simulink model "simulation_finale"  (R2017a)
settings: Solver=VariableStepAuto  StartTime=0.0  StopTime=1  RelTol=1e-2
InitFcn:
  | variable
values from neighbouring files (symbols this model uses):
  A = (pi*D^2)/4    (= 0.125663706144)    [variable.m]
  a_char_z = 0    [variable.m]
  a_cible_x = 3    [variable.m]
  a_cible_y = 4    [variable.m]
  a_cible_z = 2.22637    [variable.m]
  alpha_phi = pi/4    (= 0.785398163397)    [variable.m]
  alpha_theta = 0    [variable.m]
  Cd = 0.15    [variable.m]
  Cl = 0.05    [variable.m]
  D = 0.4    [variable.m]
  Fc = (294/0.1)*m    (= 14700)    [variable.m]
  g = 9.81    [variable.m]
  m = 5    [variable.m]
  pos_ini_char_z = 0    [variable.m]
  pos_ini_cible_x = 5    [variable.m]
  pos_ini_cible_y = 8    [variable.m]
  pos_ini_cible_z = 5    [variable.m]
  r_missile_canon = 2    [variable.m]
  rho = 1.225    [variable.m]
  v_ini_char_z = 0    [variable.m]
  v_ini_cible_x = 4    [variable.m]
  v_ini_cible_y = 2    [variable.m]
  v_ini_cible_z = 10    [variable.m]
  viscosite = 1.57*10^-5    (= 1.57e-05)    [variable.m]
  w_ini_phi = 1    [variable.m]
  w_ini_theta = 1    [variable.m]
undefined symbols (not defined in the file or in its folder): a_char_x, a_char_y, magnitude, phi_ini_canon, pos_ini_char_x, pos_ini_char_y, theta_ini_canon, v_ini_char_x, v_ini_char_y
settings Model: Creator=stabm1  LastModifiedBy=ahamm2

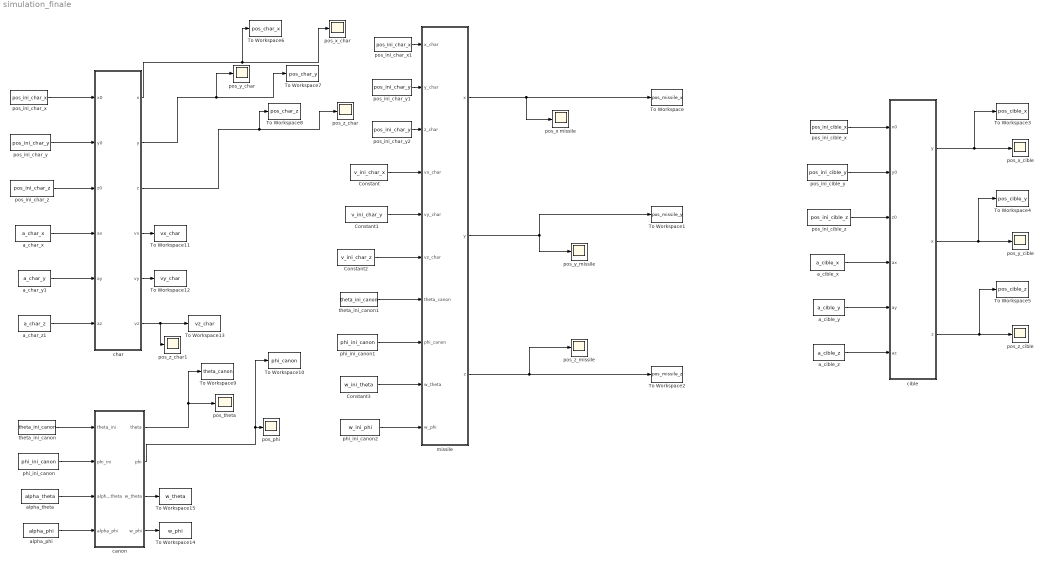
== system simulation_finale ==
  Constant : Constant  Value=v_ini_char_x
  Constant1 : Constant  Value=v_ini_char_y
  Constant2 : Constant  Value=v_ini_char_z
  Constant3 : Constant  Value=w_ini_theta
  To Workspace : ToWorkspace  VariableName=pos_missile_x  SaveFormat=Timeseries  SampleTime=-1
  To Workspace1 : ToWorkspace  VariableName=pos_missile_y  SaveFormat=Timeseries  SampleTime=-1
  To Workspace10 : ToWorkspace  VariableName=phi_canon  SaveFormat=Timeseries  SampleTime=-1
  To Workspace11 : ToWorkspace  VariableName=vx_char  SaveFormat=Timeseries  SampleTime=-1
  To Workspace12 : ToWorkspace  VariableName=vy_char  SaveFormat=Timeseries  SampleTime=-1
  To Workspace13 : ToWorkspace  VariableName=vz_char  SaveFormat=Timeseries  SampleTime=-1
  To Workspace14 : ToWorkspace  VariableName=w_phi  SaveFormat=Timeseries  SampleTime=-1
  To Workspace15 : ToWorkspace  VariableName=w_theta  SaveFormat=Timeseries  SampleTime=-1
  To Workspace2 : ToWorkspace  VariableName=pos_missile_z  SaveFormat=Timeseries  SampleTime=-1
  To Workspace3 : ToWorkspace  VariableName=pos_cible_x  SaveFormat=Timeseries  SampleTime=-1
  To Workspace4 : ToWorkspace  VariableName=pos_cible_y  SaveFormat=Timeseries  SampleTime=-1
  To Workspace5 : ToWorkspace  VariableName=pos_cible_z  SaveFormat=Timeseries  SampleTime=-1
  To Workspace6 : ToWorkspace  VariableName=pos_char_x  SaveFormat=Timeseries  SampleTime=-1
  To Workspace7 : ToWorkspace  VariableName=pos_char_y  SaveFormat=Timeseries  SampleTime=-1
  To Workspace8 : ToWorkspace  VariableName=pos_char_z  SaveFormat=Timeseries  SampleTime=-1
  To Workspace9 : ToWorkspace  VariableName=theta_canon  SaveFormat=Timeseries  SampleTime=-1
  a_char_x : Constant  Value=a_char_x
  a_char_y1 : Constant  Value=a_char_y
  a_char_z1 : Constant  Value=a_char_z
  a_cible_x : Constant  Value=a_cible_x
  a_cible_y : Constant  Value=a_cible_y
  a_cible_z : Constant  Value=a_cible_z
  alpha_phi : Constant  Value=alpha_phi
  alpha_theta : Constant  Value=alpha_theta
  canon : Subsystem  TreatAsAtomicUnit=on
  char : Subsystem  TreatAsAtomicUnit=on
  cible : Subsystem  TreatAsAtomicUnit=on
  missile : Subsystem  TreatAsAtomicUnit=on
  phi_ini_canon : Constant  Value=phi_ini_canon
  phi_ini_canon1 : Constant  Value=phi_ini_canon
  phi_ini_canon2 : Constant  Value=w_ini_phi
  pos_ini_char_x : Constant  Value=pos_ini_char_x
  pos_ini_char_x1 : Constant  Value=pos_ini_char_x
  pos_ini_char_y : Constant  Value=pos_ini_char_y
  pos_ini_char_y1 : Constant  Value=pos_ini_char_y
  pos_ini_char_y2 : Constant  Value=pos_ini_char_y
  pos_ini_char_z : Constant  Value=pos_ini_char_z
  pos_ini_cible_x : Constant  Value=pos_ini_cible_x
  pos_ini_cible_y : Constant  Value=pos_ini_cible_y
  pos_ini_cible_z : Constant  Value=pos_ini_cible_z
  pos_phi : Scope
  pos_theta : Scope
  pos_x missile : Scope
  pos_x_char : Scope
  pos_x_cible : Scope
  pos_y_char : Scope
  pos_y_cible : Scope
  pos_y_missile : Scope
  pos_z_char : Scope
  pos_z_char1 : Scope
  pos_z_cible : Scope
  pos_z_missile : Scope
  theta_ini_canon : Constant  Value=theta_ini_canon
  theta_ini_canon1 : Constant  Value=theta_ini_canon
  wires:
  a_char_y1/1 -> char/5(ay)
  a_char_z1/1 -> char/6(az)
  a_char_x/1 -> char/4(ax)
  a_cible_y/1 -> cible/5(ay)
  cible/1(y) -> To Workspace3/1, pos_x_cible/1
  a_cible_x/1 -> cible/4(ax)
  a_cible_z/1 -> cible/6(az)
  pos_ini_cible_z/1 -> cible/3(z0)
  pos_ini_cible_y/1 -> cible/2(y0)
  cible/3(z) -> To Workspace5/1, pos_z_cible/1
  pos_ini_cible_x/1 -> cible/1(x0)
  cible/2(x) -> To Workspace4/1, pos_y_cible/1
  theta_ini_canon/1 -> canon/1(theta_ini)
  alpha_phi/1 -> canon/4(alpha_phi)
  alpha_theta/1 -> canon/3(alpha_theta)
  phi_ini_canon/1 -> canon/2(phi_ini)
  missile/1(x) -> To Workspace/1, pos_x missile/1
  missile/2(y) -> To Workspace1/1, pos_y_missile/1
  missile/3(z) -> pos_z_missile/1, To Workspace2/1
  char/1(x) -> pos_x_char/1, To Workspace6/1
  char/2(y) -> pos_y_char/1, To Workspace7/1
  char/3(z) -> To Workspace8/1, pos_z_char/1
  canon/1(theta) -> pos_theta/1, To Workspace9/1
  canon/2(phi) -> pos_phi/1, To Workspace10/1
  pos_ini_char_x/1 -> char/1(x0)
  pos_ini_char_y/1 -> char/2(y0)
  pos_ini_char_z/1 -> char/3(z0)
  pos_ini_char_x1/1 -> missile/1(x_char)
  pos_ini_char_y1/1 -> missile/2(y_char)
  pos_ini_char_y2/1 -> missile/3(z_char)
  Constant/1 -> missile/4(vx_char)
  Constant1/1 -> missile/5(vy_char)
  Constant2/1 -> missile/6(vz_char)
  char/4(vx) -> To Workspace11/1
  char/5(vy) -> To Workspace12/1
  char/6(vz) -> pos_z_char1/1, To Workspace13/1
  theta_ini_canon1/1 -> missile/7(theta_canon)
  phi_ini_canon1/1 -> missile/8(phi_canon)
  Constant3/1 -> missile/9(w_theta)
  phi_ini_canon2/1 -> missile/10(w_phi)
  canon/3(w_theta) -> To Workspace15/1
  canon/4(w_phi) -> To Workspace14/1

== system simulation_finale/canon ==
  theta_ini : Inport
  phi_ini : Inport  Port=2
  alpha_theta : Inport  Port=3
  alpha_phi : Inport  Port=4
  angle_theta : Subsystem  TreatAsAtomicUnit=on
  angle_theta1 : Subsystem  TreatAsAtomicUnit=on
  theta : Outport
  phi : Outport  Port=2
  w_theta : Outport  Port=3
  w_phi : Outport  Port=4
  wires:
  theta_ini/1 -> angle_theta/1(theta_ini)
  alpha_theta/1 -> angle_theta/2(alpha_theta)
  angle_theta/1(theta) -> theta/1
  angle_theta1/1(phi) -> phi/1
  alpha_phi/1 -> angle_theta1/2(alpha_phi)
  phi_ini/1 -> angle_theta1/1(phi_ini)
  angle_theta1/2(w_phi) -> w_phi/1
  angle_theta/2(w_theta) -> w_theta/1

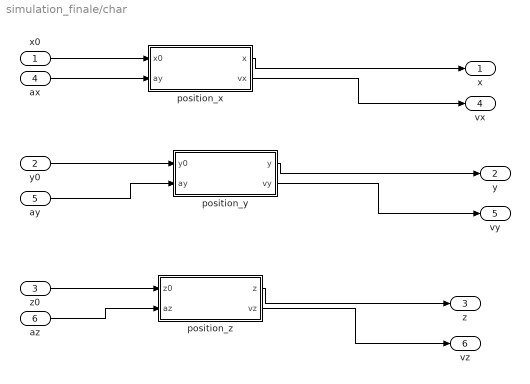
== system simulation_finale/char ==
  x0 : Inport
  y0 : Inport  Port=2
  z0 : Inport  Port=3
  ax : Inport  Port=4
  ay : Inport  Port=5
  az : Inport  Port=6
  position_x : Subsystem  TreatAsAtomicUnit=on
  position_y : Subsystem  TreatAsAtomicUnit=on
  position_z : Subsystem  TreatAsAtomicUnit=on
  x : Outport
  y : Outport  Port=2
  z : Outport  Port=3
  vx : Outport  Port=4
  vy : Outport  Port=5
  vz : Outport  Port=6
  wires:
  x0/1 -> position_x/1(x0)
  ax/1 -> position_x/2(ay)
  position_x/1(x) -> x/1
  y0/1 -> position_y/1(y0)
  ay/1 -> position_y/2(ay)
  position_y/1(y) -> y/1
  z0/1 -> position_z/1(z0)
  az/1 -> position_z/2(az)
  position_z/1(z) -> z/1
  position_x/2(vx) -> vx/1
  position_y/2(vy) -> vy/1
  position_z/2(vz) -> vz/1

== system simulation_finale/cible ==
  note: r = r0+v*t+at^2
  x0 : Inport
  y0 : Inport  Port=2
  z0 : Inport  Port=3
  ax : Inport  Port=4
  ay : Inport  Port=5
  az : Inport  Port=6
  position_x : Subsystem  TreatAsAtomicUnit=on
  position_y : Subsystem  TreatAsAtomicUnit=on
  position_z : Subsystem  TreatAsAtomicUnit=on
  y : Outport
  x : Outport  Port=2
  z : Outport  Port=3
  wires:
  x0/1 -> position_x/1(x0)
  ax/1 -> position_x/2(ay)
  position_x/1(x) -> x/1
  y0/1 -> position_y/1(y0)
  ay/1 -> position_y/2(ay)
  position_y/1(y) -> y/1
  z0/1 -> position_z/1(z0)
  az/1 -> position_z/2(az)
  position_z/1(z) -> z/1

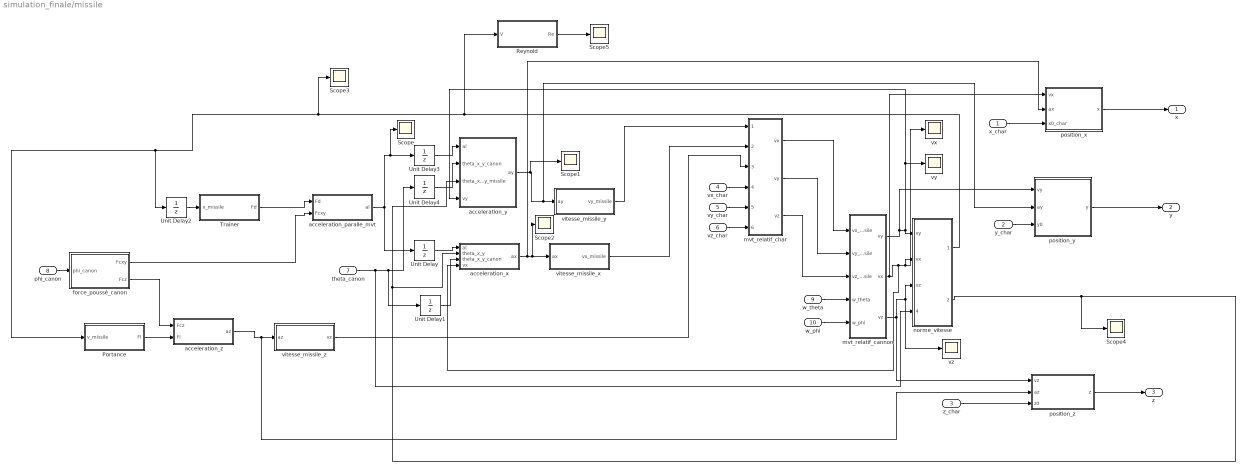
== system simulation_finale/missile ==
  x_char : Inport
  y_char : Inport  Port=2
  z_char : Inport  Port=3
  vx_char : Inport  Port=4
  vy_char : Inport  Port=5
  vz_char : Inport  Port=6
  theta_canon : Inport  Port=7
  phi_canon : Inport  Port=8
  w_theta : Inport  Port=9
  w_phi : Inport  Port=10
  Portance : Subsystem  TreatAsAtomicUnit=on
  Reynold : Subsystem  TreatAsAtomicUnit=on
  Scope{,1..5} (6 alike) : Scope
  Trainer : Subsystem  TreatAsAtomicUnit=on
  Unit Delay{,1..4} (5 alike) : UnitDelay  SampleTime=-1
  acceleration_paralle_mvt : Subsystem  TreatAsAtomicUnit=on
  acceleration_x : Subsystem  TreatAsAtomicUnit=on
  acceleration_y : Subsystem  TreatAsAtomicUnit=on
  acceleration_z : Subsystem  TreatAsAtomicUnit=on
  force_poussé_canon : Subsystem  TreatAsAtomicUnit=on
  mvt_relatif_cannon : Subsystem  TreatAsAtomicUnit=on
  mvt_relatif_char : Subsystem  TreatAsAtomicUnit=on
  "norme_vitesse " : Subsystem  TreatAsAtomicUnit=on
  position_x : Subsystem  TreatAsAtomicUnit=on
  position_y : Subsystem  TreatAsAtomicUnit=on
  position_z : Subsystem  TreatAsAtomicUnit=on
  vitesse_missile_x : Subsystem  TreatAsAtomicUnit=on
  vitesse_missile_y : Subsystem  TreatAsAtomicUnit=on
  vitesse_missile_z : Subsystem  TreatAsAtomicUnit=on
  vx : Scope
  vy : Scope
  vz : Scope
  x : Outport
  y : Outport  Port=2
  z : Outport  Port=3
  wires:
  Trainer/1(Fd) -> acceleration_paralle_mvt/1(Fd)
  Portance/1(Fl) -> acceleration_z/2(Fl)
  acceleration_paralle_mvt/1(al) -> Scope/1, Unit Delay3/1, Unit Delay/1
  "norme_vitesse "/1(v_missile) -> Reynold/1(V), Scope3/1, Unit Delay2/1, Portance/1(v_missile)
  Unit Delay/1 -> acceleration_x/1(al)
  Unit Delay2/1 -> Trainer/1(v_missile)
  Unit Delay3/1 -> acceleration_y/1(al)
  Unit Delay4/1 -> acceleration_y/2(theta_x_y_canon)
  phi_canon/1 -> force_poussé_canon/1(phi_canon)
  force_poussé_canon/2(Fcz) -> acceleration_z/1(Fcz)
  force_poussé_canon/1(Fcxy) -> acceleration_paralle_mvt/2(Fcxy)
  mvt_relatif_cannon/3(vz) -> position_z/1(vz), vz/1, "norme_vitesse "/3(vz)
  mvt_relatif_cannon/1(vy) -> position_y/1(vy), acceleration_y/4(vy), vy/1, "norme_vitesse "/1(vy)
  vitesse_missile_z/1(vz) -> mvt_relatif_char/3(vz_missile)
  position_y/1(y) -> y/1
  position_z/1(z) -> z/1
  position_x/1(x) -> x/1
  z_char/1 -> position_z/3(z0)
  x_char/1 -> position_x/3(x0_char)
  y_char/1 -> position_y/3(y0)
  vitesse_missile_y/1(vy_missile) -> mvt_relatif_char/1(vy_missile)
  acceleration_z/1(az) -> position_z/2(az), vitesse_missile_z/1(az)
  vx_char/1 -> mvt_relatif_char/4(vx_char)
  vy_char/1 -> mvt_relatif_char/5(vy_char)
  vz_char/1 -> mvt_relatif_char/6(vz_char)
  vitesse_missile_x/1(vx_missile) -> mvt_relatif_char/2(vx_missile)
  w_theta/1 -> mvt_relatif_cannon/4(w_theta)
  w_phi/1 -> mvt_relatif_cannon/5(w_phi)
  mvt_relatif_char/3(vz) -> mvt_relatif_cannon/3(vz_missile)
  mvt_relatif_char/2(vy) -> mvt_relatif_cannon/2(vy_missile)
  mvt_relatif_char/1(vx) -> mvt_relatif_cannon/1(vx_missile)
  "norme_vitesse "/2(theta_x_y) -> Scope4/1, acceleration_x/2(theta_x_y), acceleration_y/3(theta_x_y_missile)
  Unit Delay1/1 -> acceleration_x/3(theta_x_y_canon)
  theta_canon/1 -> "norme_vitesse "/4(theta_canon), Unit Delay1/1, Unit Delay4/1
  Reynold/1(Re) -> Scope5/1
  acceleration_x/1(ax) -> vitesse_missile_x/1(ax), Scope2/1, position_x/2(ax)
  acceleration_y/1(ay) -> Scope1/1, position_y/2(ay), vitesse_missile_y/1(ay)
  mvt_relatif_cannon/2(vx) -> acceleration_x/4(vx), vx/1, "norme_vitesse "/2(vx), position_x/1(vx)

== system simulation_finale/canon/angle_theta ==
  theta_ini : Inport
  alpha_theta : Inport  Port=2
  Add : Sum
  Add1 : Sum
  Clock : Clock
  Gain : Gain  Gain=1/2
  Math Function : Math  Operator=magnitude^2  SaturateOnIntegerOverflow=on
  Product : Product
  Product1 : Product
  v : Integrator  InitialCondition=w_ini_theta
  theta : Outport
  w_theta : Outport  Port=2
  wires:
  Add1/1 -> theta/1
  Math Function/1 -> Product1/1
  Product/1 -> Add/2
  Add/1 -> Add1/1
  alpha_theta/1 -> Product1/2, v/1
  Clock/1 -> Math Function/1, Product/2
  theta_ini/1 -> Add/1
  Gain/1 -> Add1/2
  Product1/1 -> Gain/1
  v/1 -> w_theta/1, Product/1

== system simulation_finale/canon/angle_theta1 ==
  phi_ini : Inport
  alpha_phi : Inport  Port=2
  Add : Sum
  Add1 : Sum
  Clock : Clock
  Gain : Gain  Gain=1/2
  Math Function : Math  Operator=magnitude^2  SaturateOnIntegerOverflow=on
  Product : Product
  Product1 : Product
  v : Integrator  InitialCondition=w_ini_phi
  phi : Outport
  w_phi : Outport  Port=2
  wires:
  Add1/1 -> phi/1
  Math Function/1 -> Product1/1
  Product/1 -> Add/2
  Add/1 -> Add1/1
  alpha_phi/1 -> Product1/2, v/1
  Clock/1 -> Math Function/1, Product/2
  phi_ini/1 -> Add/1
  Gain/1 -> Add1/2
  Product1/1 -> Gain/1
  v/1 -> w_phi/1, Product/1

== system simulation_finale/char/position_x ==
  x0 : Inport
  ay : Inport  Port=2
  Add : Sum
  Add1 : Sum
  Clock : Clock
  Gain : Gain  Gain=1/2
  Math Function : Math  Operator=magnitude^2  SaturateOnIntegerOverflow=on
  Product : Product
  Product1 : Product
  v : Integrator  InitialCondition=v_ini_char_x
  x : Outport
  vx : Outport  Port=2
  wires:
  v/1 -> vx/1, Product/1
  Product/1 -> Add/2
  Math Function/1 -> Product1/1
  Add/1 -> Add1/1
  Product1/1 -> Gain/1
  Gain/1 -> Add1/2
  Clock/1 -> Math Function/1, Product/2
  x0/1 -> Add/1
  ay/1 -> Product1/2, v/1
  Add1/1 -> x/1

== system simulation_finale/char/position_y ==
  y0 : Inport
  ay : Inport  Port=2
  Add : Sum
  Add1 : Sum
  Clock : Clock
  Gain : Gain  Gain=1/2
  Math Function : Math  Operator=magnitude^2  SaturateOnIntegerOverflow=on
  Product : Product
  Product1 : Product
  v : Integrator  InitialCondition=v_ini_char_y
  y : Outport
  vy : Outport  Port=2
  wires:
  v/1 -> vy/1, Product/1
  Product/1 -> Add/2
  Math Function/1 -> Product1/1
  Add/1 -> Add1/1
  Product1/1 -> Gain/1
  Gain/1 -> Add1/2
  Clock/1 -> Math Function/1, Product/2
  y0/1 -> Add/1
  ay/1 -> Product1/2, v/1
  Add1/1 -> y/1

== system simulation_finale/char/position_z ==
  z0 : Inport
  az : Inport  Port=2
  Add : Sum
  Add1 : Sum
  Clock : Clock
  Gain : Gain  Gain=1/2
  Math Function : Math  Operator=magnitude^2  SaturateOnIntegerOverflow=on
  Product : Product
  Product1 : Product
  v : Integrator  InitialCondition=v_ini_char_z
  z : Outport
  vz : Outport  Port=2
  wires:
  v/1 -> Product/1, vz/1
  Product/1 -> Add/2
  Math Function/1 -> Product1/1
  Add/1 -> Add1/1
  Product1/1 -> Gain/1
  Gain/1 -> Add1/2
  Clock/1 -> Math Function/1, Product/2
  z0/1 -> Add/1
  az/1 -> Product1/2, v/1
  Add1/1 -> z/1

== system simulation_finale/cible/position_x ==
  x0 : Inport
  ay : Inport  Port=2
  Add : Sum
  Add1 : Sum
  Clock : Clock
  Gain : Gain  Gain=1/2
  Math Function : Math  Operator=magnitude^2  SaturateOnIntegerOverflow=on
  Product : Product
  Product1 : Product
  v : Integrator  InitialCondition=v_ini_cible_x
  x : Outport
  wires:
  v/1 -> Product/1
  Product/1 -> Add/2
  Math Function/1 -> Product1/1
  Add/1 -> Add1/1
  Product1/1 -> Gain/1
  Gain/1 -> Add1/2
  Clock/1 -> Math Function/1, Product/2
  x0/1 -> Add/1
  ay/1 -> Product1/2, v/1
  Add1/1 -> x/1

== system simulation_finale/cible/position_y ==
  y0 : Inport
  ay : Inport  Port=2
  Add : Sum
  Add1 : Sum
  Clock : Clock
  Gain : Gain  Gain=1/2
  Math Function : Math  Operator=magnitude^2  SaturateOnIntegerOverflow=on
  Product : Product
  Product1 : Product
  v : Integrator  InitialCondition=v_ini_cible_y
  y : Outport
  wires:
  v/1 -> Product/1
  Product/1 -> Add/2
  Math Function/1 -> Product1/1
  Add/1 -> Add1/1
  Product1/1 -> Gain/1
  Gain/1 -> Add1/2
  Clock/1 -> Math Function/1, Product/2
  y0/1 -> Add/1
  ay/1 -> Product1/2, v/1
  Add1/1 -> y/1

== system simulation_finale/cible/position_z ==
  z0 : Inport
  az : Inport  Port=2
  Add : Sum
  Add1 : Sum
  Clock : Clock
  Gain : Gain  Gain=1/2
  Math Function : Math  Operator=magnitude^2  SaturateOnIntegerOverflow=on
  Product : Product
  Product1 : Product
  v : Integrator  InitialCondition=v_ini_cible_z
  z : Outport
  wires:
  v/1 -> Product/1
  Product/1 -> Add/2
  Math Function/1 -> Product1/1
  Add/1 -> Add1/1
  Product1/1 -> Gain/1
  Gain/1 -> Add1/2
  Clock/1 -> Math Function/1, Product/2
  z0/1 -> Add/1
  az/1 -> Product1/2, v/1
  Add1/1 -> z/1

== system simulation_finale/missile/Portance ==
  v_missile : Inport
  Constant : Constant  Value=Cl
  Gain : Gain  Gain=0.5*rho*A
  Math Function : Math  Operator=magnitude^2  SaturateOnIntegerOverflow=on
  Product : Product
  Fl : Outport
  wires:
  Product/1 -> Fl/1
  Gain/1 -> Product/1
  Constant/1 -> Product/2
  v_missile/1 -> Math Function/1
  Math Function/1 -> Gain/1

== system simulation_finale/missile/Reynold ==
  V : Inport
  Gain : Gain  Gain=D/viscosite
  To Workspace : ToWorkspace  VariableName=Re  SaveFormat=Timeseries  SampleTime=-1
  Re : Outport
  wires:
  V/1 -> Gain/1
  Gain/1 -> Re/1, To Workspace/1

== system simulation_finale/missile/Trainer ==
  v_missile : Inport
  Constant : Constant  Value=Cd
  Gain : Gain  Gain=0.5*rho*A
  Math Function : Math  Operator=magnitude^2  SaturateOnIntegerOverflow=on
  Product : Product
  Fd : Outport
  wires:
  v_missile/1 -> Math Function/1
  Math Function/1 -> Gain/1
  Gain/1 -> Product/1
  Constant/1 -> Product/2
  Product/1 -> Fd/1

== system simulation_finale/missile/acceleration_paralle_mvt ==
  Fd : Inport
  Fcxy : Inport  Port=2
  Add : Sum  Inputs=-+
  Gain : Gain  Gain=1/m
  al : Outport
  wires:
  Gain/1 -> al/1
  Add/1 -> Gain/1
  Fcxy/1 -> Add/2
  Fd/1 -> Add/1

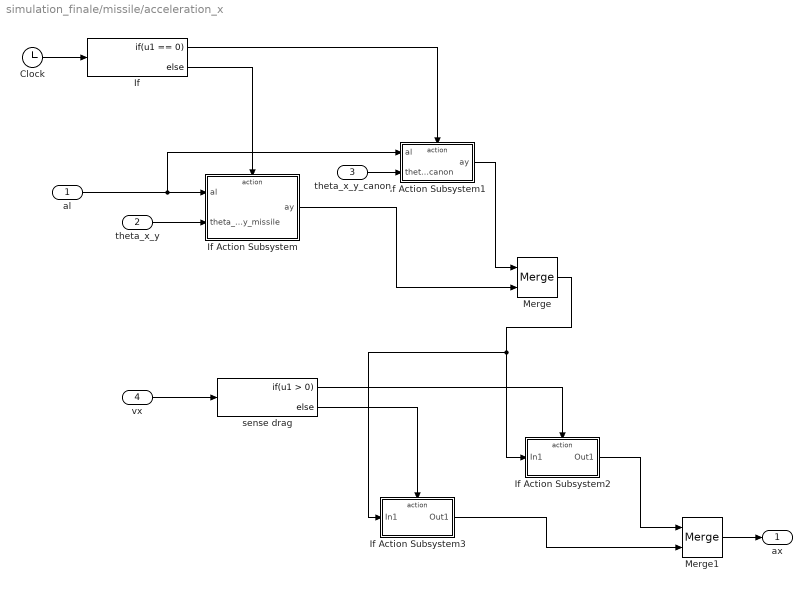
== system simulation_finale/missile/acceleration_x ==
  al : Inport
  theta_x_y : Inport  Port=2
  theta_x_y_canon : Inport  Port=3
  vx : Inport  Port=4
  Clock : Clock
  If : If  IfExpression=u1 == 0
  If Action Subsystem : Subsystem  TreatAsAtomicUnit=on
  If Action Subsystem1 : Subsystem  TreatAsAtomicUnit=on
  If Action Subsystem2 : Subsystem  TreatAsAtomicUnit=on
  If Action Subsystem3 : Subsystem  TreatAsAtomicUnit=on
  Merge : Merge
  Merge1 : Merge
  sense drag : If  ZeroCross=off
  ax : Outport
  wires:
  If/1 -> If Action Subsystem1/Action
  theta_x_y/1 -> If Action Subsystem/2(theta_x_y_missile)
  If Action Subsystem/1(ay) -> Merge/2
  If/2 -> If Action Subsystem/Action
  theta_x_y_canon/1 -> If Action Subsystem1/2(theta_canon)
  Clock/1 -> If/1
  al/1 -> If Action Subsystem1/1(al), If Action Subsystem/1(al)
  If Action Subsystem1/1(ay) -> Merge/1
  sense drag/1 -> If Action Subsystem2/Action
  sense drag/2 -> If Action Subsystem3/Action
  Merge1/1 -> ax/1
  If Action Subsystem2/1(Out1) -> Merge1/1
  If Action Subsystem3/1(Out1) -> Merge1/2
  Merge/1 -> If Action Subsystem3/1(In1), If Action Subsystem2/1(In1)
  vx/1 -> sense drag/1

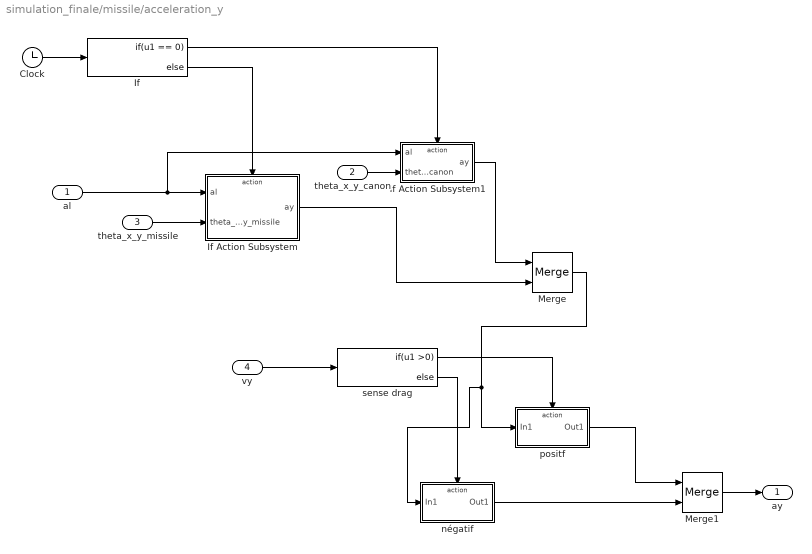
== system simulation_finale/missile/acceleration_y ==
  al : Inport
  theta_x_y_canon : Inport  Port=2
  theta_x_y_missile : Inport  Port=3
  vy : Inport  Port=4
  Clock : Clock
  If : If  IfExpression=u1 == 0
  If Action Subsystem : Subsystem  TreatAsAtomicUnit=on
  If Action Subsystem1 : Subsystem  TreatAsAtomicUnit=on
  Merge : Merge
  Merge1 : Merge
  négatif : Subsystem  TreatAsAtomicUnit=on
  positf : Subsystem  TreatAsAtomicUnit=on
  sense drag : If  IfExpression=u1 >0  ZeroCross=off
  ay : Outport
  wires:
  If/1 -> If Action Subsystem1/Action
  If/2 -> If Action Subsystem/Action
  Clock/1 -> If/1
  If Action Subsystem1/1(ay) -> Merge/1
  al/1 -> If Action Subsystem1/1(al), If Action Subsystem/1(al)
  theta_x_y_canon/1 -> If Action Subsystem1/2(theta_canon)
  If Action Subsystem/1(ay) -> Merge/2
  theta_x_y_missile/1 -> If Action Subsystem/2(theta_x_y_missile)
  vy/1 -> sense drag/1
  Merge1/1 -> ay/1
  sense drag/1 -> positf/Action
  sense drag/2 -> négatif/Action
  Merge/1 -> négatif/1(In1), positf/1(In1)
  positf/1(Out1) -> Merge1/1
  négatif/1(Out1) -> Merge1/2

== system simulation_finale/missile/acceleration_z ==
  Fcz : Inport
  Fl : Inport  Port=2
  Add : Sum  Inputs=++-
  Constant : Constant  Value=m*g
  Gain : Gain  Gain=1/m
  Scope : Scope
  Scope1 : Scope
  Scope2 : Scope
  az : Outport
  wires:
  Fl/1 -> Scope/1, Add/1
  Add/1 -> Gain/1
  Gain/1 -> az/1
  Constant/1 -> Scope1/1, Add/3
  Fcz/1 -> Scope2/1, Add/2

== system simulation_finale/missile/force_poussé_canon ==
  phi_canon : Inport
  Clock : Clock
  If : If  IfExpression=u1 ==0  ZeroCross=off
  Merge : Merge
  Merge1 : Merge
  pas de poussé : Subsystem  TreatAsAtomicUnit=on
  poussé du canon : Subsystem  TreatAsAtomicUnit=on
  Fcxy : Outport
  Fcz : Outport  Port=2
  wires:
  Clock/1 -> If/1
  Merge/1 -> Fcz/1
  Merge1/1 -> Fcxy/1
  If/1 -> poussé du canon/Action
  phi_canon/1 -> poussé du canon/1(phi_canon)
  poussé du canon/1(Fcz) -> Merge/1
  poussé du canon/2(Fcxy) -> Merge1/1
  If/2 -> pas de poussé/Action
  pas de poussé/1(pas_de_pousse) -> Merge/2
  pas de poussé/2(pas_de_pousse2) -> Merge1/2

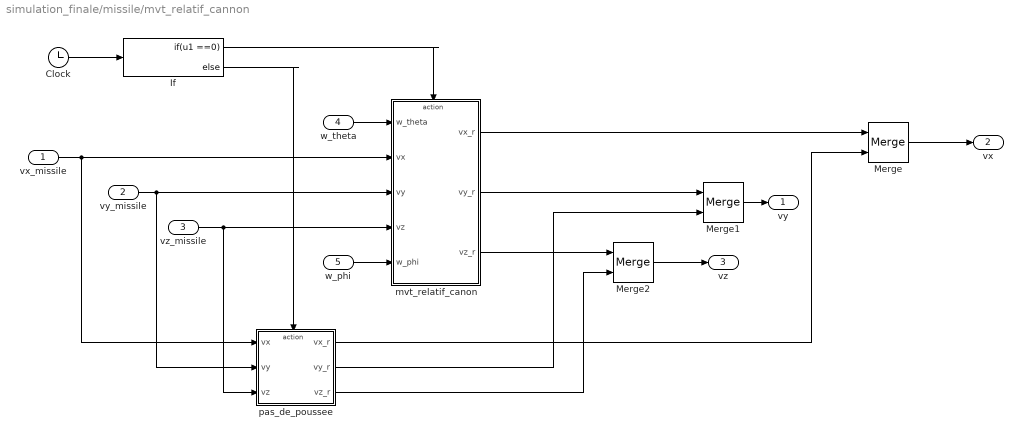
== system simulation_finale/missile/mvt_relatif_cannon ==
  vx_missile : Inport
  vy_missile : Inport  Port=2
  vz_missile : Inport  Port=3
  w_theta : Inport  Port=4
  w_phi : Inport  Port=5
  Clock : Clock
  If : If  IfExpression=u1 ==0
  Merge : Merge
  Merge1 : Merge
  Merge2 : Merge
  mvt_relatif_canon : Subsystem  TreatAsAtomicUnit=on
  pas_de_poussee : Subsystem  TreatAsAtomicUnit=on
  vy : Outport
  vx : Outport  Port=2
  vz : Outport  Port=3
  wires:
  If/1 -> mvt_relatif_canon/Action
  If/2 -> pas_de_poussee/Action
  Merge/1 -> vx/1
  Merge1/1 -> vy/1
  Merge2/1 -> vz/1
  w_theta/1 -> mvt_relatif_canon/1(w_theta)
  vy_missile/1 -> mvt_relatif_canon/3(vy), pas_de_poussee/2(vy)
  mvt_relatif_canon/1(vx_r) -> Merge/1
  mvt_relatif_canon/2(vy_r) -> Merge1/1
  mvt_relatif_canon/3(vz_r) -> Merge2/1
  vx_missile/1 -> mvt_relatif_canon/2(vx), pas_de_poussee/1(vx)
  vz_missile/1 -> pas_de_poussee/3(vz), mvt_relatif_canon/4(vz)
  w_phi/1 -> mvt_relatif_canon/5(w_phi)
  pas_de_poussee/1(vx_r) -> Merge/2
  pas_de_poussee/2(vy_r) -> Merge1/2
  pas_de_poussee/3(vz_r) -> Merge2/2
  Clock/1 -> If/1

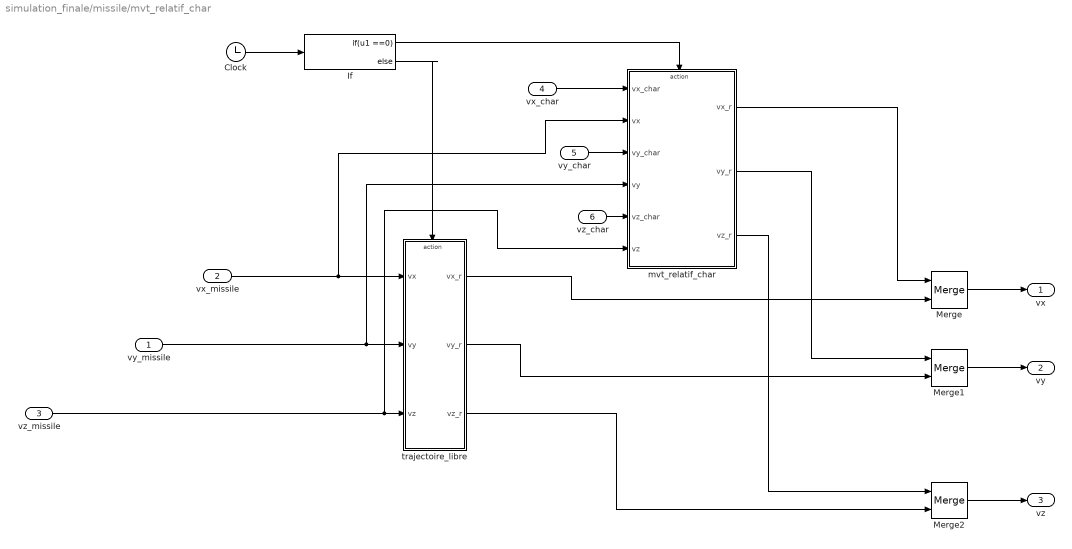
== system simulation_finale/missile/mvt_relatif_char ==
  vy_missile : Inport
  vx_missile : Inport  Port=2
  vz_missile : Inport  Port=3
  vx_char : Inport  Port=4
  vy_char : Inport  Port=5
  vz_char : Inport  Port=6
  Clock : Clock
  If : If  IfExpression=u1 ==0
  Merge : Merge
  Merge1 : Merge
  Merge2 : Merge
  mvt_relatif_char : Subsystem  TreatAsAtomicUnit=on
  trajectoire_libre : Subsystem  TreatAsAtomicUnit=on
  vx : Outport
  vy : Outport  Port=2
  vz : Outport  Port=3
  wires:
  Clock/1 -> If/1
  If/1 -> mvt_relatif_char/Action
  If/2 -> trajectoire_libre/Action
  mvt_relatif_char/1(vx_r) -> Merge/1
  trajectoire_libre/1(vx_r) -> Merge/2
  mvt_relatif_char/2(vy_r) -> Merge1/1
  trajectoire_libre/2(vy_r) -> Merge1/2
  mvt_relatif_char/3(vz_r) -> Merge2/1
  trajectoire_libre/3(vz_r) -> Merge2/2
  Merge/1 -> vx/1
  Merge1/1 -> vy/1
  Merge2/1 -> vz/1
  vx_missile/1 -> mvt_relatif_char/2(vx), trajectoire_libre/1(vx)
  vx_char/1 -> mvt_relatif_char/1(vx_char)
  vy_char/1 -> mvt_relatif_char/3(vy_char)
  vy_missile/1 -> mvt_relatif_char/4(vy), trajectoire_libre/2(vy)
  vz_char/1 -> mvt_relatif_char/5(vz_char)
  vz_missile/1 -> mvt_relatif_char/6(vz), trajectoire_libre/3(vz)

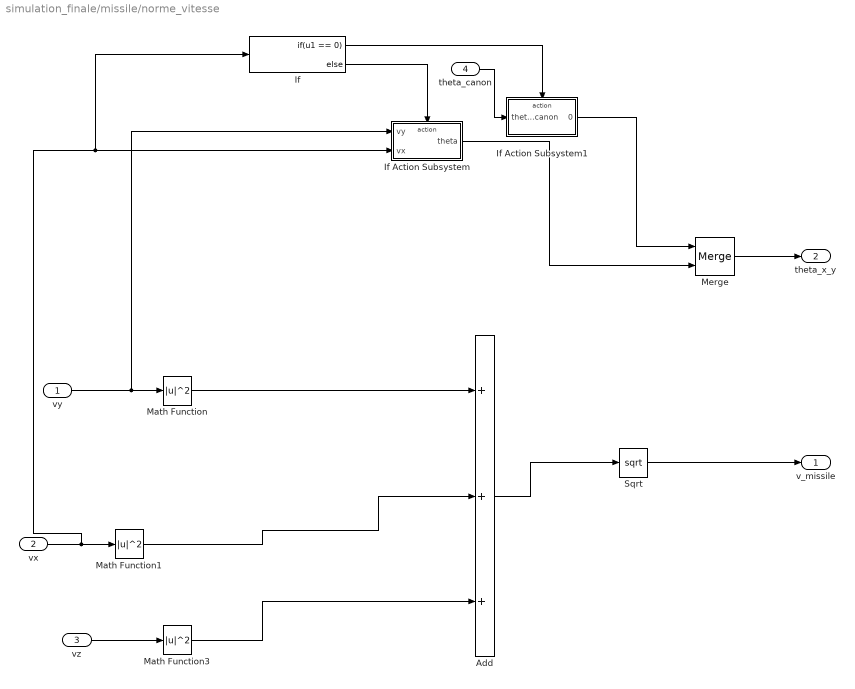
== system simulation_finale/missile/norme_vitesse  ==
  vy : Inport
  vx : Inport  Port=2
  vz : Inport  Port=3
  theta_canon : Inport  Port=4
  Add : Sum  Inputs=+++
  If : If  IfExpression=u1 == 0
  If Action Subsystem : Subsystem  TreatAsAtomicUnit=on
  If Action Subsystem1 : Subsystem  TreatAsAtomicUnit=on
  Math Function : Math  Operator=magnitude^2  SaturateOnIntegerOverflow=on
  Math Function1 : Math  Operator=magnitude^2  SaturateOnIntegerOverflow=on
  Math Function3 : Math  Operator=magnitude^2  SaturateOnIntegerOverflow=on
  Merge : Merge
  Sqrt : Sqrt  SaturateOnIntegerOverflow=on
  v_missile : Outport
  theta_x_y : Outport  Port=2
  wires:
  vy/1 -> If Action Subsystem/1(vy), Math Function/1
  vz/1 -> Math Function3/1
  Math Function/1 -> Add/1
  Math Function3/1 -> Add/3
  Add/1 -> Sqrt/1
  Sqrt/1 -> v_missile/1
  Math Function1/1 -> Add/2
  vx/1 -> If/1, If Action Subsystem/2(vx), Math Function1/1
  If/1 -> If Action Subsystem1/Action
  If/2 -> If Action Subsystem/Action
  Merge/1 -> theta_x_y/1
  If Action Subsystem1/1(0) -> Merge/1
  If Action Subsystem/1(theta) -> Merge/2
  theta_canon/1 -> If Action Subsystem1/1(theta_canon)

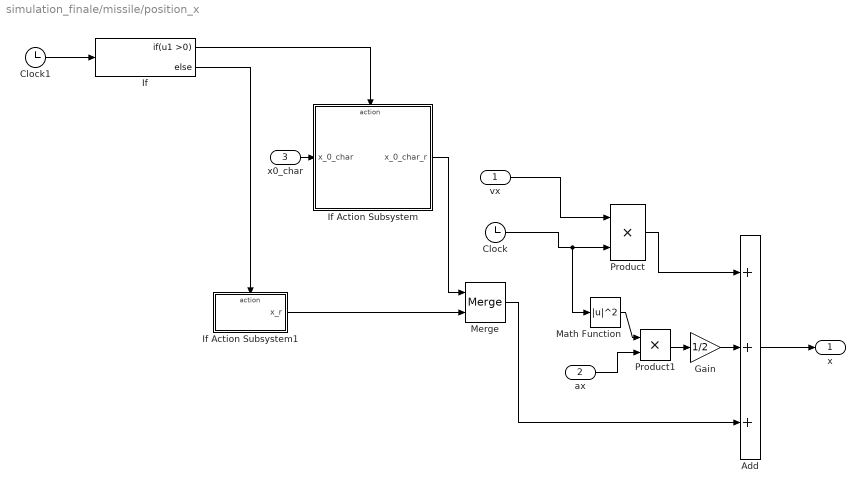
== system simulation_finale/missile/position_x ==
  vx : Inport
  ax : Inport  Port=2
  x0_char : Inport  Port=3
  Add : Sum  Inputs=+++
  Clock : Clock
  Clock1 : Clock
  Gain : Gain  Gain=1/2
  If : If  IfExpression=u1 >0
  If Action Subsystem : Subsystem  TreatAsAtomicUnit=on
  If Action Subsystem1 : Subsystem  TreatAsAtomicUnit=on
  Math Function : Math  Operator=magnitude^2  SaturateOnIntegerOverflow=on
  Merge : Merge
  Product : Product
  Product1 : Product
  x : Outport
  wires:
  vx/1 -> Product/1
  Clock/1 -> Math Function/1, Product/2
  Product/1 -> Add/1
  Math Function/1 -> Product1/1
  ax/1 -> Product1/2
  Gain/1 -> Add/2
  Product1/1 -> Gain/1
  If/1 -> If Action Subsystem/Action
  If/2 -> If Action Subsystem1/Action
  Add/1 -> x/1
  x0_char/1 -> If Action Subsystem/1(x_0_char)
  If Action Subsystem/1(x_0_char_r) -> Merge/1
  Merge/1 -> Add/3
  Clock1/1 -> If/1
  If Action Subsystem1/1(x_r) -> Merge/2

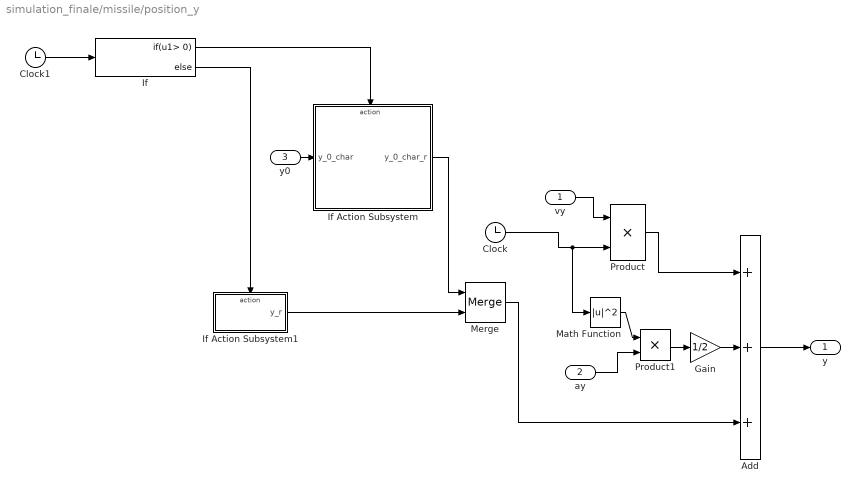
== system simulation_finale/missile/position_y ==
  vy : Inport
  ay : Inport  Port=2
  y0 : Inport  Port=3
  Add : Sum  Inputs=+++
  Clock : Clock
  Clock1 : Clock
  Gain : Gain  Gain=1/2
  If : If  IfExpression=u1> 0
  If Action Subsystem : Subsystem  TreatAsAtomicUnit=on
  If Action Subsystem1 : Subsystem  TreatAsAtomicUnit=on
  Math Function : Math  Operator=magnitude^2  SaturateOnIntegerOverflow=on
  Merge : Merge
  Product : Product
  Product1 : Product
  y : Outport
  wires:
  Merge/1 -> Add/3
  Add/1 -> y/1
  Clock/1 -> Math Function/1, Product/2
  If Action Subsystem/1(y_0_char_r) -> Merge/1
  If/2 -> If Action Subsystem1/Action
  If/1 -> If Action Subsystem/Action
  Gain/1 -> Add/2
  Product1/1 -> Gain/1
  If Action Subsystem1/1(y_r) -> Merge/2
  ay/1 -> Product1/2
  Clock1/1 -> If/1
  Math Function/1 -> Product1/1
  Product/1 -> Add/1
  vy/1 -> Product/1
  y0/1 -> If Action Subsystem/1(y_0_char)

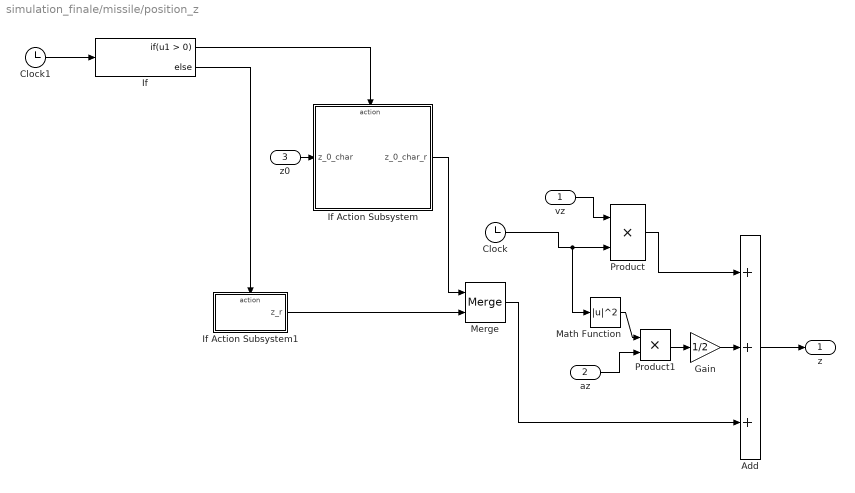
== system simulation_finale/missile/position_z ==
  vz : Inport
  az : Inport  Port=2
  z0 : Inport  Port=3
  Add : Sum  Inputs=+++
  Clock : Clock
  Clock1 : Clock
  Gain : Gain  Gain=1/2
  If : If
  If Action Subsystem : Subsystem  TreatAsAtomicUnit=on
  If Action Subsystem1 : Subsystem  TreatAsAtomicUnit=on
  Math Function : Math  Operator=magnitude^2  SaturateOnIntegerOverflow=on
  Merge : Merge
  Product : Product
  Product1 : Product
  z : Outport
  wires:
  z0/1 -> If Action Subsystem/1(z_0_char)
  Product1/1 -> Gain/1
  Gain/1 -> Add/2
  If/1 -> If Action Subsystem/Action
  If/2 -> If Action Subsystem1/Action
  Clock/1 -> Math Function/1, Product/2
  If Action Subsystem/1(z_0_char_r) -> Merge/1
  Merge/1 -> Add/3
  Clock1/1 -> If/1
  If Action Subsystem1/1(z_r) -> Merge/2
  Add/1 -> z/1
  Product/1 -> Add/1
  vz/1 -> Product/1
  Math Function/1 -> Product1/1
  az/1 -> Product1/2

== system simulation_finale/missile/vitesse_missile_x ==
  ax : Inport
  v : Integrator
  vx_missile : Outport
  wires:
  ax/1 -> v/1
  v/1 -> vx_missile/1

== system simulation_finale/missile/vitesse_missile_y ==
  ay : Inport
  v : Integrator
  vy_missile : Outport
  wires:
  v/1 -> vy_missile/1
  ay/1 -> v/1

== system simulation_finale/missile/vitesse_missile_z ==
  az : Inport
  v : Integrator
  vz : Outport
  wires:
  v/1 -> vz/1
  az/1 -> v/1

== system simulation_finale/missile/acceleration_x/If Action Subsystem ==
  al : Inport
  theta_x_y_missile : Inport  Port=2
  Action Port : ActionPort  ActionType=else
  Product : Product
  Trigonometric Function : Trigonometry  Operator=cos
  ay : Outport
  wires:
  theta_x_y_missile/1 -> Trigonometric Function/1
  Trigonometric Function/1 -> Product/2
  al/1 -> Product/1
  Product/1 -> ay/1

== system simulation_finale/missile/acceleration_x/If Action Subsystem1 ==
  al : Inport
  theta_canon : Inport  Port=2
  Action Port : ActionPort  ActionType=then
  Product : Product
  Trigonometric Function : Trigonometry  Operator=cos
  ay : Outport
  wires:
  al/1 -> Product/1
  Product/1 -> ay/1
  Trigonometric Function/1 -> Product/2
  theta_canon/1 -> Trigonometric Function/1

== system simulation_finale/missile/acceleration_x/If Action Subsystem2 ==
  In1 : Inport
  Action Port : ActionPort  ActionType=then
  Out1 : Outport
  wires:
  In1/1 -> Out1/1

== system simulation_finale/missile/acceleration_x/If Action Subsystem3 ==
  In1 : Inport
  Action Port : ActionPort  ActionType=else
  Gain : Gain  Gain=-1
  Out1 : Outport
  wires:
  Gain/1 -> Out1/1
  In1/1 -> Gain/1

== system simulation_finale/missile/acceleration_y/If Action Subsystem ==
  al : Inport
  theta_x_y_missile : Inport  Port=2
  Action Port : ActionPort  ActionType=else
  Product : Product
  Trigonometric Function : Trigonometry
  ay : Outport
  wires:
  theta_x_y_missile/1 -> Trigonometric Function/1
  Trigonometric Function/1 -> Product/2
  al/1 -> Product/1
  Product/1 -> ay/1

== system simulation_finale/missile/acceleration_y/If Action Subsystem1 ==
  al : Inport
  theta_canon : Inport  Port=2
  Action Port : ActionPort  ActionType=then
  Product : Product
  Trigonometric Function : Trigonometry
  ay : Outport
  wires:
  al/1 -> Product/1
  Product/1 -> ay/1
  Trigonometric Function/1 -> Product/2
  theta_canon/1 -> Trigonometric Function/1

== system simulation_finale/missile/acceleration_y/négatif ==
  In1 : Inport
  Action Port : ActionPort  ActionType=else
  Gain : Gain  Gain=-1
  Out1 : Outport
  wires:
  Gain/1 -> Out1/1
  In1/1 -> Gain/1

== system simulation_finale/missile/acceleration_y/positf ==
  In1 : Inport
  Action Port : ActionPort  ActionType=then
  Out1 : Outport
  wires:
  In1/1 -> Out1/1

== system simulation_finale/missile/force_poussé_canon/pas de poussé ==
  Action Port : ActionPort  ActionType=else
  Constant : Constant  Value=0
  pas_de_pousse : Outport
  pas_de_pousse2 : Outport  Port=2
  wires:
  Constant/1 -> pas_de_pousse2/1, pas_de_pousse/1

== system simulation_finale/missile/force_poussé_canon/poussé du canon ==
  phi_canon : Inport
  Action Port : ActionPort  ActionType=then
  Constant : Constant  Value=Fc
  Product : Product
  Product1 : Product
  Scope1 : Scope
  Trigonometric Function : Trigonometry  Operator=cos
  Trigonometric Function1 : Trigonometry
  Fcz : Outport
  Fcxy : Outport  Port=2
  wires:
  Trigonometric Function/1 -> Product1/1
  phi_canon/1 -> Trigonometric Function/1, Trigonometric Function1/1
  Product1/1 -> Fcxy/1
  Trigonometric Function1/1 -> Scope1/1, Product/2
  Constant/1 -> Product/1, Product1/2
  Product/1 -> Fcz/1

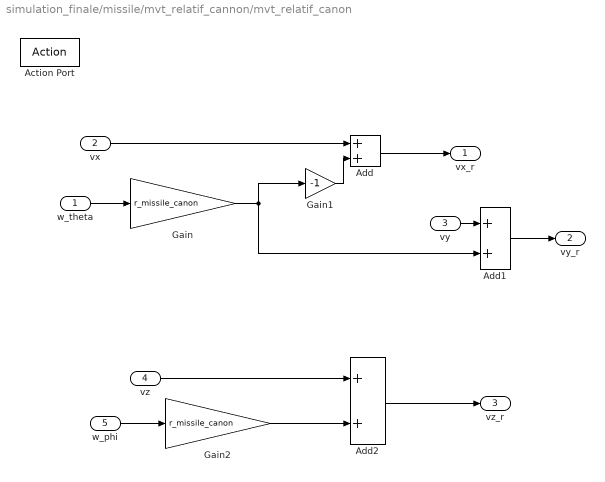
== system simulation_finale/missile/mvt_relatif_cannon/mvt_relatif_canon ==
  w_theta : Inport
  vx : Inport  Port=2
  vy : Inport  Port=3
  vz : Inport  Port=4
  w_phi : Inport  Port=5
  Action Port : ActionPort  ActionType=then
  Add : Sum
  Add1 : Sum
  Add2 : Sum
  Gain : Gain  Gain=r_missile_canon
  Gain1 : Gain  Gain=-1
  Gain2 : Gain  Gain=r_missile_canon
  vx_r : Outport
  vy_r : Outport  Port=2
  vz_r : Outport  Port=3
  wires:
  Gain1/1 -> Add/2
  Gain/1 -> Gain1/1, Add1/2
  vx/1 -> Add/1
  w_theta/1 -> Gain/1
  Add/1 -> vx_r/1
  vy/1 -> Add1/1
  Add1/1 -> vy_r/1
  Add2/1 -> vz_r/1
  Gain2/1 -> Add2/2
  vz/1 -> Add2/1
  w_phi/1 -> Gain2/1

== system simulation_finale/missile/mvt_relatif_cannon/pas_de_poussee ==
  vx : Inport
  vy : Inport  Port=2
  vz : Inport  Port=3
  Action Port : ActionPort  ActionType=else
  vx_r : Outport
  vy_r : Outport  Port=2
  vz_r : Outport  Port=3
  wires:
  vx/1 -> vx_r/1
  vy/1 -> vy_r/1
  vz/1 -> vz_r/1

== system simulation_finale/missile/mvt_relatif_char/mvt_relatif_char ==
  vx_char : Inport
  vx : Inport  Port=2
  vy_char : Inport  Port=3
  vy : Inport  Port=4
  vz_char : Inport  Port=5
  vz : Inport  Port=6
  Action Port : ActionPort  ActionType=then
  Add : Sum
  Add1 : Sum
  Add2 : Sum
  vx_r : Outport
  vy_r : Outport  Port=2
  vz_r : Outport  Port=3
  wires:
  vx_char/1 -> Add/1
  vx/1 -> Add/2
  vy_char/1 -> Add1/1
  vy/1 -> Add1/2
  vz_char/1 -> Add2/1
  vz/1 -> Add2/2
  Add/1 -> vx_r/1
  Add1/1 -> vy_r/1
  Add2/1 -> vz_r/1

== system simulation_finale/missile/mvt_relatif_char/trajectoire_libre ==
  vx : Inport
  vy : Inport  Port=2
  vz : Inport  Port=3
  Action Port : ActionPort  ActionType=else
  vx_r : Outport
  vy_r : Outport  Port=2
  vz_r : Outport  Port=3
  wires:
  vx/1 -> vx_r/1
  vy/1 -> vy_r/1
  vz/1 -> vz_r/1

== system simulation_finale/missile/norme_vitesse /If Action Subsystem ==
  vy : Inport
  vx : Inport  Port=2
  Action Port : ActionPort  ActionType=else
  Divide : Product  Inputs=*/
  Trigonometric Function : Trigonometry  Operator=atan
  theta : Outport
  wires:
  Divide/1 -> Trigonometric Function/1
  Trigonometric Function/1 -> theta/1
  vx/1 -> Divide/2
  vy/1 -> Divide/1

== system simulation_finale/missile/norme_vitesse /If Action Subsystem1 ==
  theta_canon : Inport
  Action Port : ActionPort  ActionType=then
  0 : Outport
  wires:
  theta_canon/1 -> 0/1

== system simulation_finale/missile/position_x/If Action Subsystem ==
  x_0_char : Inport
  Action Port : ActionPort  ActionType=then
  x_0_char_r : Outport
  wires:
  x_0_char/1 -> x_0_char_r/1

== system simulation_finale/missile/position_x/If Action Subsystem1 ==
  Action Port : ActionPort  ActionType=else
  Constant : Constant  Value=pi
  x_r : Outport
  wires:
  Constant/1 -> x_r/1

== system simulation_finale/missile/position_y/If Action Subsystem ==
  y_0_char : Inport
  Action Port : ActionPort  ActionType=then
  y_0_char_r : Outport
  wires:
  y_0_char/1 -> y_0_char_r/1

== system simulation_finale/missile/position_y/If Action Subsystem1 ==
  Action Port : ActionPort  ActionType=else
  Constant : Constant  Value=pi
  y_r : Outport
  wires:
  Constant/1 -> y_r/1

== system simulation_finale/missile/position_z/If Action Subsystem ==
  z_0_char : Inport
  Action Port : ActionPort  ActionType=then
  z_0_char_r : Outport
  wires:
  z_0_char/1 -> z_0_char_r/1

== system simulation_finale/missile/position_z/If Action Subsystem1 ==
  Action Port : ActionPort  ActionType=else
  Constant : Constant  Value=pi
  z_r : Outport
  wires:
  Constant/1 -> z_r/1
